simulink library "AEMS_Standard_Library"  (R2016b)
settings: Solver=ode45  StartTime=0.0  StopTime=10.0  RelTol=1e-3
undefined symbols (not defined in the file or in its folder): BkPY, carto, Cbx_extegr, Cbx_lpegrsys, Cbx_portegr, Cnx_bnk_nr_conf, Cnx_cyl_nr_conf, ConfigManagement, configuration_management, Cxx_dcm_io_tmr_end_xxxx, Cxx_dcm_rt_tmr_end, Cxx_DID_xxxx_IO_max, Cxx_DID_xxxx_IO_min, Cxx_egrhsofs, Cxx_vmaniegi, DEM_DEBOUNCE_FREEZE, DEM_DTR_CTL_INVISIBLE, DEM_DTR_CTL_NORMAL, Dem_DtrId2_XXX, Dem_DtrId3_XXX, Dem_DtrId4_XXX, Dem_DtrId5_XXX, Dem_DtrId6_XXX, Dem_DtrId7_XXX, Dem_DtrId8_XXX, Dem_DtrId9_XXX, Dem_DtrId_XXX, Dem_EnableConditionId2_XXX, Dem_EnableConditionId3_XXX, Dem_EnableConditionId4_XXX, Dem_EnableConditionId5_XXX, Dem_EnableConditionId6_XXX, Dem_EnableConditionId7_XXX, Dem_EnableConditionId8_XXX, Dem_EnableConditionId_XXX, Dem_EventId, Dem_EventId2_XXX, Dem_EventId3_XXX, Dem_EventId4_XXX, Dem_EventId5_XXX, Dem_EventId6_XXX, Dem_EventId7_XXX, Dem_EventId8_XXX, Dem_EventId9_XXX, Dem_EventId_Device_Faulttype, Dem_EventId_XXX, DEM_IUMPR_GENERAL_DENOMINATOR, DEM_OPCYC_IGNITION, Dem_RatioId2_XXX, Dem_RatioId3_XXX, Dem_RatioId4_XXX, Dem_RatioId5_XXX, Dem_RatioId6_XXX, Dem_RatioId7_XXX, Dem_RatioId8_XXX, Dem_RatioId_XXX, Dem_StorageConditionId2_XXX, Dem_StorageConditionId3_XXX, Dem_StorageConditionId4_XXX, Dem_StorageConditionId5_XXX ... (+65)
libraries: AEMS_Standard_Library x477, simulink x2
(part 27 of 39)

== system AEMS_Standard_Library/DISCONTINUITIES/AEMS_MULTI_PORT_TIME_SWITCH/pulse_and_old ==
  Vsx_sel : Inport  Tag=AM,In,0,1,Name,C;CMP,Port,PortWidth,SampleTime;
  AEMS_UNITDELAY_EXTERNALIC : AEMS_Standard_Library/DISCRETE/AEMS_UNITDELAY_EXTERNALIC  Tag=[LIB]
      settings: AttributesFormatString=%<MaskType>
  Relational_Operator : RelationalOperator  Tag=AM,Std,2,1;CMP,Operator;  Operator=~=  OutDataTypeStr=boolean  RndMeth=Nearest  InputSameDT=on
  Switch : Switch  Tag=GEN,Threshold;AM,Switch,2,1;CMP,Threshold;  Criteria=u2 ~= 0  RndMeth=Zero  SaturateOnIntegerOverflow=on  InputSameDT=on
      settings: AttributesFormatString=Criteria=%<Criteria>
  Unit_Delay : UnitDelay  Tag=GEN,X0,SampleTime;AM,Std,1,1;CMP,X0,SampleTime;  InitialCondition=1  SampleTime=-1
      settings: AttributesFormatString=IC = %<X0>
  Vbx_sel_puls : Outport  Tag=AM,Out,1,0,Name,NC;CMP,Port,OutputWhenDisabled,InitialOutput;
  Vsx_sel_old : Outport  Tag=AM,Out,1,0,Name,NC;CMP,Port,OutputWhenDisabled,InitialOutput;  Port=2
  wires:
  Unit_Delay/1 -> Switch/3
  Switch/1 -> Unit_Delay/1, Vsx_sel_old/1
  Relational_Operator/1 -> Switch/2, Vbx_sel_puls/1
  Vsx_sel/1 -> AEMS_UNITDELAY_EXTERNALIC/1, AEMS_UNITDELAY_EXTERNALIC/2, Relational_Operator/2
  AEMS_UNITDELAY_EXTERNALIC/1 -> Switch/1, Relational_Operator/1

== system AEMS_Standard_Library/DISCONTINUITIES/AEMS_MULTI_PORT_TIME_SWITCH/slop_on ==
  Vxx_swi_trs : Inport  Tag=AM,In,0,1,Name,C;CMP,Port,PortWidth,SampleTime;
  Vbx_sel_puls : Inport  Tag=AM,In,0,1,Name,C;CMP,Port,PortWidth,SampleTime;  Port=2
  Constant3 : Constant  Tag=AM,Constant,0,1,Value;CMP,Value;  OutDataTypeStr=Inherit: Inherit via back propagation
  Relational_Operator4 : RelationalOperator  Tag=AM,Std,2,1;CMP,Operator;  OutDataTypeStr=boolean  RndMeth=Nearest  InputSameDT=on
  SR_FlipFlop1 : Subsystem
  Terminator : Terminator
      settings: Tag=AM,Nothing;
  Vbx_slop_on : Outport  Tag=AM,Out,1,0,Name,NC;CMP,Port,OutputWhenDisabled,InitialOutput;
  wires:
  SR_FlipFlop1/2(QNot) -> Terminator/1
  SR_FlipFlop1/1(Q) -> Vbx_slop_on/1
  Vxx_swi_trs/1 -> Relational_Operator4/1
  Vbx_sel_puls/1 -> SR_FlipFlop1/1(S)
  Constant3/1 -> Relational_Operator4/2
  Relational_Operator4/1 -> SR_FlipFlop1/2(R)

== system AEMS_Standard_Library/DISCONTINUITIES/AEMS_MULTI_PORT_TIME_SWITCH/transient_timer ==
  Vxx_swi_t : Inport  Tag=AM,In,0,1,Name,C;CMP,Port,PortWidth,SampleTime;
  Vbx_sel_puls : Inport  Tag=AM,In,0,1,Name,C;CMP,Port,PortWidth,SampleTime;  Port=2
  dT : Inport  Tag=AM,In,0,1,Name,C;CMP,Port,PortWidth,SampleTime;  Port=3
  AEMS_DIVISION_BY_ZERO : Subsystem
  Constant1 : Constant  Tag=AM,Constant,0,1,Value;CMP,Value;  OutDataTypeStr=Inherit: Inherit via back propagation
  Constant2 : Constant  Tag=AM,Constant,0,1,Value;CMP,Value;  OutDataTypeStr=Inherit: Inherit via back propagation
  Constant4 : Constant  Tag=AM,Constant,0,1,Value;CMP,Value;  OutDataTypeStr=Inherit: Inherit via back propagation
  Relational_Operator3 : RelationalOperator  Tag=AM,Std,2,1;CMP,Operator;  OutDataTypeStr=boolean  RndMeth=Nearest  InputSameDT=on
  Sum : Sum  Tag=AM,Std,Inputs,1;CMP,Inputs;  OutDataTypeStr=Inherit: Inherit via back propagation  RndMeth=Zero  InputSameDT=on
  Switch : Switch  Tag=GEN,Threshold;AM,Switch,2,1;CMP,Threshold;  Criteria=u2 ~= 0  RndMeth=Zero  SaturateOnIntegerOverflow=on  InputSameDT=on
      settings: AttributesFormatString=Criteria=%<Criteria>
  Switch1 : Switch  Tag=GEN,Threshold;AM,Switch,2,1;CMP,Threshold;  Criteria=u2 ~= 0  RndMeth=Zero  SaturateOnIntegerOverflow=on  InputSameDT=on
      settings: AttributesFormatString=Criteria=%<Criteria>
  Unit_Delay1 : UnitDelay  Tag=GEN,X0,SampleTime;AM,Std,1,1;CMP,X0,SampleTime;  SampleTime=-1
      settings: AttributesFormatString=IC = %<X0>
  Vxx_swi_trs : Outport  Tag=AM,Out,1,0,Name,NC;CMP,Port,OutputWhenDisabled,InitialOutput;
  wires:
  Unit_Delay1/1 -> Sum/2, Relational_Operator3/1
  AEMS_DIVISION_BY_ZERO/1(ans) -> Sum/1, Switch/1
  Vbx_sel_puls/1 -> Switch/2
  Switch/1 -> Unit_Delay1/1, Vxx_swi_trs/1
  Sum/1 -> Switch1/3
  Switch1/1 -> Switch/3
  Constant1/1 -> Relational_Operator3/2
  Relational_Operator3/1 -> Switch1/2
  Constant2/1 -> Switch1/1
  Constant4/1 -> AEMS_DIVISION_BY_ZERO/3(ans_of_0div)
  dT/1 -> AEMS_DIVISION_BY_ZERO/2(num)
  Vxx_swi_t/1 -> AEMS_DIVISION_BY_ZERO/1(den)

== system AEMS_Standard_Library/DISCONTINUITIES/AEMS_SLEW_RATE/Slew_rate ==
  MAX_SLEW_RATE : Inport
  INPUT : Inport  Port=2
  MIN_SLEW_RATE : Inport  Port=3
  Constant1 : Constant  Value=true
  Slewing : Subsystem
  Switch : Switch  Criteria=u2 ~= 0  RndMeth=Zero  SaturateOnIntegerOverflow=on  InputSameDT=on
      settings: AttributesFormatString=Criteria=%<Criteria>
  UnitDelay : UnitDelay  SampleTime=-1
      settings: AttributesFormatString=IC = %<X0>
  UnitDelay1 : UnitDelay  InitialCondition=false  SampleTime=-1
      settings: AttributesFormatString=IC = %<X0>
  OUTPUT : Outport
  wires:
  MAX_SLEW_RATE/1 -> Slewing/2(MAX_SLEW_RATE)
  Switch/1 -> UnitDelay/1, OUTPUT/1
  INPUT/1 -> Slewing/4(INPUT), Switch/3
  Slewing/1(OUTPUT) -> Switch/1
  MIN_SLEW_RATE/1 -> Slewing/3(MIN_SLEW_RATE)
  Constant1/1 -> UnitDelay1/1
  UnitDelay/1 -> Slewing/1(OUTPUT_Prev)
  UnitDelay1/1 -> Switch/2

== system AEMS_Standard_Library/DISCONTINUITIES/AEMS_SLOPE_SWITCH/Signal_Change_Compute ==
  Switch_Cmd : Inport
  Relational_Operator : RelationalOperator  Operator=~=  OutDataTypeStr=boolean  RndMeth=Nearest  InputSameDT=on
  UnitDelay : UnitDelay  SampleTime=-1
      settings: AttributesFormatString=IC = %<X0>
  Signal_Change : Outport
  wires:
  Relational_Operator/1 -> Signal_Change/1
  Switch_Cmd/1 -> Relational_Operator/1, UnitDelay/1
  UnitDelay/1 -> Relational_Operator/2

== system AEMS_Standard_Library/DISCONTINUITIES/AEMS_SLOPE_SWITCH/Slope_On_Block ==
  Signal_Change : Inport  Tag=AM,In,0,1,Name,C;CMP,Port,PortWidth,SampleTime;
  Input : Inport  Tag=AM,In,0,1,Name,C;CMP,Port,PortWidth,SampleTime;  Port=2
  Pos_Slope : Inport  Tag=AM,In,0,1,Name,C;CMP,Port,PortWidth,SampleTime;  Port=3
  Neg_Slope : Inport  Tag=AM,In,0,1,Name,C;CMP,Port,PortWidth,SampleTime;  Port=4
  Prev_Output : Inport  Port=5
  Enable_Slope_On_Block : EnablePort
      settings: AttributesFormatString=StatesWhenEnabling: %<StatesWhenEnabling>
  Error_Due_To_High_Slope_Test : Subsystem
  Output_Comparision : Subsystem
  Output_Not_Equals_Input : Outport  Tag=AM,Out,1,0,Name,NC;CMP,Port,OutputWhenDisabled,InitialOutput;
  Output : Outport  Tag=AM,Out,1,0,Name,NC;CMP,Port,OutputWhenDisabled,InitialOutput;  Port=2
  wires:
  Error_Due_To_High_Slope_Test/1(Test_passed) -> Output_Comparision/1(Test_passed)
  Neg_Slope/1 -> Output_Comparision/5(Neg_Slope)
  Input/1 -> Output_Comparision/2(Input)
  Pos_Slope/1 -> Output_Comparision/3(Pos_Slope)
  Prev_Output/1 -> Output_Comparision/4(Prev_Output)
  Output_Comparision/2(Output) -> Output/1
  Output_Comparision/1(Output_Not_Equals_Input) -> Output_Not_Equals_Input/1
  Output_Comparision/3(RelOp2_out) -> Error_Due_To_High_Slope_Test/2(Output_Less_Than_Input)
  Output_Comparision/4(RelOp1_out) -> Error_Due_To_High_Slope_Test/3(Output_Greater_Than_Input)
  Signal_Change/1 -> Error_Due_To_High_Slope_Test/1(Signal_Change)

== system AEMS_Standard_Library/DISCONTINUITIES/AEMS_SLOPE_SWITCH/Slope_On_Compute ==
  Signal_Change : Inport  Tag=AM,In,0,1,Name,C;CMP,Port,PortWidth,SampleTime;
  Output_Not_Equals_Input : Inport  Tag=AM,In,0,1,Name,C;CMP,Port,PortWidth,SampleTime;  Port=2
  Constant1 : Constant  Value=false
  Constant3 : Constant  Value=true
  LogicalOperator : Logic  Operator=OR  OutDataTypeStr=boolean
  Switch2 : Switch  Tag=GEN,Threshold;AM,Switch,2,1;CMP,Threshold;  Criteria=u2 ~= 0  RndMeth=Zero  SaturateOnIntegerOverflow=on  InputSameDT=on
      settings: AttributesFormatString=Criteria=%<Criteria>
  UnitDelay1 : UnitDelay  InitialCondition=false  SampleTime=-1
      settings: AttributesFormatString=IC = %<X0>
  Slope_On : Outport  Tag=AM,Out,1,0,Name,NC;CMP,Port,OutputWhenDisabled,InitialOutput;
  wires:
  Switch2/1 -> LogicalOperator/2
  Constant1/1 -> Switch2/3
  Constant3/1 -> UnitDelay1/1
  UnitDelay1/1 -> Switch2/2
  Signal_Change/1 -> Switch2/1
  LogicalOperator/1 -> Slope_On/1
  Output_Not_Equals_Input/1 -> LogicalOperator/1

== system AEMS_Standard_Library/DISCONTINUITIES/AEMS_SLOPE_SWITCH_3INPUTS/Signal_Change_Compute ==
  Switch_Cmd : Inport
  Relational_Operator : RelationalOperator  Operator=~=  OutDataTypeStr=boolean  RndMeth=Nearest  InputSameDT=on
  UnitDelay : UnitDelay  SampleTime=-1
      settings: AttributesFormatString=IC = %<X0>
  Signal_Change : Outport
  wires:
  UnitDelay/1 -> Relational_Operator/2
  Switch_Cmd/1 -> UnitDelay/1, Relational_Operator/1
  Relational_Operator/1 -> Signal_Change/1

== system AEMS_Standard_Library/DISCONTINUITIES/AEMS_SLOPE_SWITCH_3INPUTS/Slope_On_Block ==
  Signal_Change : Inport  Tag=AM,In,0,1,Name,C;CMP,Port,PortWidth,SampleTime;
  Input : Inport  Tag=AM,In,0,1,Name,C;CMP,Port,PortWidth,SampleTime;  Port=2
  Pos_Slope : Inport  Tag=AM,In,0,1,Name,C;CMP,Port,PortWidth,SampleTime;  Port=3
  Neg_Slope : Inport  Tag=AM,In,0,1,Name,C;CMP,Port,PortWidth,SampleTime;  Port=4
  Prev_Output : Inport  Port=5
  Enable_Slope_On_Block : EnablePort
      settings: AttributesFormatString=StatesWhenEnabling: %<StatesWhenEnabling>
  Error_Due_To_High_Slope_Test : Subsystem
  Output_Comparision : Subsystem
  Output_Not_Equals_Input : Outport  Tag=AM,Out,1,0,Name,NC;CMP,Port,OutputWhenDisabled,InitialOutput;
  Output : Outport  Tag=AM,Out,1,0,Name,NC;CMP,Port,OutputWhenDisabled,InitialOutput;  Port=2
  wires:
  Signal_Change/1 -> Error_Due_To_High_Slope_Test/1(Signal_Change)
  Output_Comparision/4(RelOp1_out) -> Error_Due_To_High_Slope_Test/2(Output_Greater_Than_Input)
  Output_Comparision/3(RelOp2_out) -> Error_Due_To_High_Slope_Test/3(Output_Less_Than_Input)
  Output_Comparision/1(Output_Not_Equals_Input) -> Output_Not_Equals_Input/1
  Output_Comparision/2(Output) -> Output/1
  Error_Due_To_High_Slope_Test/1(Test_passed) -> Output_Comparision/1(Test_passed)
  Prev_Output/1 -> Output_Comparision/4(Prev_Output)
  Pos_Slope/1 -> Output_Comparision/3(Pos_Slope)
  Input/1 -> Output_Comparision/2(Input)
  Neg_Slope/1 -> Output_Comparision/5(Neg_Slope)

== system AEMS_Standard_Library/DISCONTINUITIES/AEMS_SLOPE_SWITCH_3INPUTS/Slope_On_Compute ==
  Signal_Change : Inport  Tag=AM,In,0,1,Name,C;CMP,Port,PortWidth,SampleTime;
  Output_Not_Equals_Input : Inport  Tag=AM,In,0,1,Name,C;CMP,Port,PortWidth,SampleTime;  Port=2
  Constant : Constant  Value=true
  Constant1 : Constant  Value=false
  Logical_Operator : Logic  Operator=OR  OutDataTypeStr=boolean
  Switch1 : Switch  Tag=GEN,Threshold;AM,Switch,2,1;CMP,Threshold;  Criteria=u2 ~= 0  RndMeth=Zero  SaturateOnIntegerOverflow=on  InputSameDT=on
      settings: AttributesFormatString=Criteria=%<Criteria>
  UnitDelay3 : UnitDelay  InitialCondition=false  SampleTime=-1
      settings: AttributesFormatString=IC = %<X0>
  Slope_On : Outport  Tag=AM,Out,1,0,Name,NC;CMP,Port,OutputWhenDisabled,InitialOutput;
  wires:
  Output_Not_Equals_Input/1 -> Logical_Operator/1
  Logical_Operator/1 -> Slope_On/1
  Constant/1 -> UnitDelay3/1
  UnitDelay3/1 -> Switch1/2
  Switch1/1 -> Logical_Operator/2
  Signal_Change/1 -> Switch1/1
  Constant1/1 -> Switch1/3

== system AEMS_Standard_Library/DISCONTINUITIES/AEMS_SLOPE_SWITCH_4INPUTS/Signal_Change_Compute ==
  Switch_Cmd : Inport
  Relational_Operator : RelationalOperator  Operator=~=  OutDataTypeStr=boolean  RndMeth=Nearest  InputSameDT=on
  UnitDelay : UnitDelay  SampleTime=-1
      settings: AttributesFormatString=IC = %<X0>
  Signal_Change : Outport
  wires:
  UnitDelay/1 -> Relational_Operator/2
  Switch_Cmd/1 -> UnitDelay/1, Relational_Operator/1
  Relational_Operator/1 -> Signal_Change/1

== system AEMS_Standard_Library/DISCONTINUITIES/AEMS_SLOPE_SWITCH_4INPUTS/Slope_On_Block ==
  Signal_Change : Inport  Tag=AM,In,0,1,Name,C;CMP,Port,PortWidth,SampleTime;
  Input : Inport  Tag=AM,In,0,1,Name,C;CMP,Port,PortWidth,SampleTime;  Port=2
  Pos_Slope : Inport  Tag=AM,In,0,1,Name,C;CMP,Port,PortWidth,SampleTime;  Port=3
  Neg_Slope : Inport  Tag=AM,In,0,1,Name,C;CMP,Port,PortWidth,SampleTime;  Port=4
  Prev_Output : Inport  Port=5
  Enable_Slope_On_Block : EnablePort
      settings: AttributesFormatString=StatesWhenEnabling: %<StatesWhenEnabling>
  Error_Due_To_High_Slope_Test : Subsystem
  Output_Comparision : Subsystem
  Output_Not_Equals_Input : Outport  Tag=AM,Out,1,0,Name,NC;CMP,Port,OutputWhenDisabled,InitialOutput;
  Output : Outport  Tag=AM,Out,1,0,Name,NC;CMP,Port,OutputWhenDisabled,InitialOutput;  Port=2
  wires:
  Signal_Change/1 -> Error_Due_To_High_Slope_Test/1(Signal_Change)
  Output_Comparision/4(RelOp1_out) -> Error_Due_To_High_Slope_Test/2(Output_Greater_Than_Input)
  Output_Comparision/3(RelOp2_out) -> Error_Due_To_High_Slope_Test/3(Output_Less_Than_Input)
  Output_Comparision/1(Output_Not_Equals_Input) -> Output_Not_Equals_Input/1
  Output_Comparision/2(Output) -> Output/1
  Error_Due_To_High_Slope_Test/1(Test_passed) -> Output_Comparision/1(Test_passed)
  Prev_Output/1 -> Output_Comparision/4(Prev_Output)
  Pos_Slope/1 -> Output_Comparision/3(Pos_Slope)
  Input/1 -> Output_Comparision/2(Input)
  Neg_Slope/1 -> Output_Comparision/5(Neg_Slope)

== system AEMS_Standard_Library/DISCONTINUITIES/AEMS_SLOPE_SWITCH_4INPUTS/Slope_On_Compute ==
  Signal_Change : Inport  Tag=AM,In,0,1,Name,C;CMP,Port,PortWidth,SampleTime;
  Output_Not_Equals_Input : Inport  Tag=AM,In,0,1,Name,C;CMP,Port,PortWidth,SampleTime;  Port=2
  Constant : Constant  Value=true
  Constant1 : Constant  Value=false
  Logical_Operator : Logic  Operator=OR  OutDataTypeStr=boolean
  Switch1 : Switch  Tag=GEN,Threshold;AM,Switch,2,1;CMP,Threshold;  Criteria=u2 ~= 0  RndMeth=Zero  SaturateOnIntegerOverflow=on  InputSameDT=on
      settings: AttributesFormatString=Criteria=%<Criteria>
  UnitDelay3 : UnitDelay  InitialCondition=false  SampleTime=-1
      settings: AttributesFormatString=IC = %<X0>
  Slope_On : Outport  Tag=AM,Out,1,0,Name,NC;CMP,Port,OutputWhenDisabled,InitialOutput;
  wires:
  Output_Not_Equals_Input/1 -> Logical_Operator/1
  Logical_Operator/1 -> Slope_On/1
  Constant/1 -> UnitDelay3/1
  UnitDelay3/1 -> Switch1/2
  Switch1/1 -> Logical_Operator/2
  Signal_Change/1 -> Switch1/1
  Constant1/1 -> Switch1/3

== system AEMS_Standard_Library/DISCONTINUITIES/AEMS_SLOPE_SWITCH_6INPUTS/Signal_Change_Compute ==
  Switch_Cmd : Inport
  Relational_Operator : RelationalOperator  Operator=~=  OutDataTypeStr=boolean  RndMeth=Nearest  InputSameDT=on
  Unit_Delay : UnitDelay  SampleTime=-1
      settings: AttributesFormatString=IC = %<X0>
  Signal_Change : Outport
  wires:
  Relational_Operator/1 -> Signal_Change/1
  Switch_Cmd/1 -> Relational_Operator/1, Unit_Delay/1
  Unit_Delay/1 -> Relational_Operator/2

== system AEMS_Standard_Library/DISCONTINUITIES/AEMS_SLOPE_SWITCH_6INPUTS/Slope_On_Block ==
  Signal_Change : Inport  Tag=AM,In,0,1,Name,C;CMP,Port,PortWidth,SampleTime;
  Input : Inport  Tag=AM,In,0,1,Name,C;CMP,Port,PortWidth,SampleTime;  Port=2
  Pos_Slope : Inport  Tag=AM,In,0,1,Name,C;CMP,Port,PortWidth,SampleTime;  Port=3
  Neg_Slope : Inport  Tag=AM,In,0,1,Name,C;CMP,Port,PortWidth,SampleTime;  Port=4
  Prev_Output : Inport  Port=5
  Enable_Slope_On_Block : EnablePort
      settings: AttributesFormatString=StatesWhenEnabling: %<StatesWhenEnabling>
  Error_Due_To_High_Slope_Test : Subsystem
  Output_Comparision : Subsystem
  Output_Not_Equals_Input : Outport  Tag=AM,Out,1,0,Name,NC;CMP,Port,OutputWhenDisabled,InitialOutput;
  Output : Outport  Tag=AM,Out,1,0,Name,NC;CMP,Port,OutputWhenDisabled,InitialOutput;  Port=2
  wires:
  Error_Due_To_High_Slope_Test/1(Test_passed) -> Output_Comparision/1(Test_passed)
  Neg_Slope/1 -> Output_Comparision/5(Neg_Slope)
  Input/1 -> Output_Comparision/2(Input)
  Pos_Slope/1 -> Output_Comparision/3(Pos_Slope)
  Prev_Output/1 -> Output_Comparision/4(Prev_Output)
  Output_Comparision/2(Output) -> Output/1
  Output_Comparision/1(Output_Not_Equals_Input) -> Output_Not_Equals_Input/1
  Output_Comparision/3(RelOp2_out) -> Error_Due_To_High_Slope_Test/2(Output_Less_Than_Input)
  Output_Comparision/4(RelOp1_out) -> Error_Due_To_High_Slope_Test/3(Output_Greater_Than_Input)
  Signal_Change/1 -> Error_Due_To_High_Slope_Test/1(Signal_Change)

== system AEMS_Standard_Library/DISCONTINUITIES/AEMS_SLOPE_SWITCH_6INPUTS/Slope_On_Compute ==
  Signal_Change : Inport  Tag=AM,In,0,1,Name,C;CMP,Port,PortWidth,SampleTime;
  Output_Not_Equals_Input : Inport  Tag=AM,In,0,1,Name,C;CMP,Port,PortWidth,SampleTime;  Port=2
  Constant : Constant  Value=true
  Constant1 : Constant  Value=false
  Logical_Operator : Logic  Operator=OR  OutDataTypeStr=boolean
  Switch1 : Switch  Tag=GEN,Threshold;AM,Switch,2,1;CMP,Threshold;  Criteria=u2 ~= 0  RndMeth=Zero  SaturateOnIntegerOverflow=on  InputSameDT=on
      settings: AttributesFormatString=Criteria=%<Criteria>
  Unit_Delay3 : UnitDelay  InitialCondition=false  SampleTime=-1
      settings: AttributesFormatString=IC = %<X0>
  Slope_On : Outport  Tag=AM,Out,1,0,Name,NC;CMP,Port,OutputWhenDisabled,InitialOutput;
  wires:
  Constant1/1 -> Switch1/3
  Signal_Change/1 -> Switch1/1
  Switch1/1 -> Logical_Operator/2
  Unit_Delay3/1 -> Switch1/2
  Constant/1 -> Unit_Delay3/1
  Logical_Operator/1 -> Slope_On/1
  Output_Not_Equals_Input/1 -> Logical_Operator/1

== system AEMS_Standard_Library/DISCONTINUITIES/AEMS_SLOPE_SWITCH_8INPUTS/Signal_Change_Compute ==
  Switch_Cmd : Inport
  Relational_Operator : RelationalOperator  Operator=~=  OutDataTypeStr=boolean  RndMeth=Nearest  InputSameDT=on
  Unit_Delay : UnitDelay  SampleTime=-1
      settings: AttributesFormatString=IC = %<X0>
  Signal_Change : Outport
  wires:
  Relational_Operator/1 -> Signal_Change/1
  Switch_Cmd/1 -> Relational_Operator/1, Unit_Delay/1
  Unit_Delay/1 -> Relational_Operator/2

== system AEMS_Standard_Library/DISCONTINUITIES/AEMS_SLOPE_SWITCH_8INPUTS/Slope_On_Block ==
  Signal_Change : Inport  Tag=AM,In,0,1,Name,C;CMP,Port,PortWidth,SampleTime;
  Input : Inport  Tag=AM,In,0,1,Name,C;CMP,Port,PortWidth,SampleTime;  Port=2
  Pos_Slope : Inport  Tag=AM,In,0,1,Name,C;CMP,Port,PortWidth,SampleTime;  Port=3
  Neg_Slope : Inport  Tag=AM,In,0,1,Name,C;CMP,Port,PortWidth,SampleTime;  Port=4
  Prev_Output : Inport  Port=5
  Enable_Slope_On_Block : EnablePort
      settings: AttributesFormatString=StatesWhenEnabling: %<StatesWhenEnabling>
  Error_Due_To_High_Slope_Test : Subsystem
  Output_Comparision : Subsystem
  Output_Not_Equals_Input : Outport  Tag=AM,Out,1,0,Name,NC;CMP,Port,OutputWhenDisabled,InitialOutput;
  Output : Outport  Tag=AM,Out,1,0,Name,NC;CMP,Port,OutputWhenDisabled,InitialOutput;  Port=2
  wires:
  Error_Due_To_High_Slope_Test/1(Test_passed) -> Output_Comparision/1(Test_passed)
  Neg_Slope/1 -> Output_Comparision/5(Neg_Slope)
  Input/1 -> Output_Comparision/2(Input)
  Pos_Slope/1 -> Output_Comparision/3(Pos_Slope)
  Prev_Output/1 -> Output_Comparision/4(Prev_Output)
  Output_Comparision/2(Output) -> Output/1
  Output_Comparision/1(Output_Not_Equals_Input) -> Output_Not_Equals_Input/1
  Output_Comparision/3(RelOp2_out) -> Error_Due_To_High_Slope_Test/2(Output_Less_Than_Input)
  Output_Comparision/4(RelOp1_out) -> Error_Due_To_High_Slope_Test/3(Output_Greater_Than_Input)
  Signal_Change/1 -> Error_Due_To_High_Slope_Test/1(Signal_Change)

== system AEMS_Standard_Library/DISCONTINUITIES/AEMS_SLOPE_SWITCH_8INPUTS/Slope_On_Compute ==
  Signal_Change : Inport  Tag=AM,In,0,1,Name,C;CMP,Port,PortWidth,SampleTime;
  Output_Not_Equals_Input : Inport  Tag=AM,In,0,1,Name,C;CMP,Port,PortWidth,SampleTime;  Port=2
  Constant : Constant  Value=true
  Constant1 : Constant  Value=false
  Logical_Operator : Logic  Operator=OR  OutDataTypeStr=boolean
  Switch1 : Switch  Tag=GEN,Threshold;AM,Switch,2,1;CMP,Threshold;  Criteria=u2 ~= 0  RndMeth=Zero  SaturateOnIntegerOverflow=on  InputSameDT=on
      settings: AttributesFormatString=Criteria=%<Criteria>
  Unit_Delay3 : UnitDelay  InitialCondition=false  SampleTime=-1
      settings: AttributesFormatString=IC = %<X0>
  Slope_On : Outport  Tag=AM,Out,1,0,Name,NC;CMP,Port,OutputWhenDisabled,InitialOutput;
  wires:
  Constant1/1 -> Switch1/3
  Signal_Change/1 -> Switch1/1
  Switch1/1 -> Logical_Operator/2
  Unit_Delay3/1 -> Switch1/2
  Constant/1 -> Unit_Delay3/1
  Logical_Operator/1 -> Slope_On/1
  Output_Not_Equals_Input/1 -> Logical_Operator/1

== system AEMS_Standard_Library/FILTER/AEMS_FILTER_WITH_DELAY_CONTROL/DivisionByZero ==
  ans_of_0div : Inport  Tag=AM,In,0,1,Name,C;CMP,Port,PortWidth,SampleTime;
  num : Inport  Tag=AM,In,0,1,Name,C;CMP,Port,PortWidth,SampleTime;  Port=2
  den : Inport  Tag=AM,In,0,1,Name,C;CMP,Port,PortWidth,SampleTime;  Port=3
  Divide : Product  Inputs=*/  OutDataTypeStr=Inherit: Inherit via back propagation  RndMeth=Zero
  MinMax1 : MinMax  Function=max  Inputs=2  OutDataTypeStr=Inherit: Inherit via back propagation  RndMeth=Zero  InputSameDT=on
  RelationalOperator : RelationalOperator  Tag=AM,Std,2,1;CMP,Operator;  Operator=~=  OutDataTypeStr=boolean  RndMeth=Nearest  InputSameDT=on
  Switch1 : Switch  Tag=GEN,Threshold;AM,Switch,2,1;CMP,Threshold;  Criteria=u2 ~= 0  RndMeth=Zero  SaturateOnIntegerOverflow=on  InputSameDT=on
      settings: AttributesFormatString=Criteria=%<Criteria>
  imm_zero : Constant  Tag=AM,Constant,0,1,Value;CMP,Value;  Value=0  OutDataTypeStr=Inherit: Inherit via back propagation
  imm_zero3 : Constant  Tag=AM,Constant,0,1,Value;CMP,Value;  Value=1.1920929e-07  OutDataTypeStr=Inherit: Inherit via back propagation
  ans : Outport  Tag=AM,Out,1,0,Name,NC;CMP,Port,OutputWhenDisabled,InitialOutput;
  wires:
  RelationalOperator/1 -> Switch1/2
  imm_zero/1 -> RelationalOperator/2
  Switch1/1 -> ans/1
  num/1 -> Divide/1
  Divide/1 -> Switch1/1
  ans_of_0div/1 -> Switch1/3
  den/1 -> RelationalOperator/1, MinMax1/2
  MinMax1/1 -> Divide/2
  imm_zero3/1 -> MinMax1/1

== system AEMS_Standard_Library/FILTER/AEMS_FILTER_WITH_DELAY_CONTROL/First_Order_Filter ==
  filter_parameter : Inport
      settings: AttributesFormatString=<tsample=%<SampleTime>>
  input : Inport  Port=2
      settings: AttributesFormatString=<tsample=%<SampleTime>>
  initial : Inport  Port=3  OutDataTypeStr=boolean
      settings: AttributesFormatString=<tsample=%<SampleTime>>
  Constant1 : Constant  OutDataTypeStr=Inherit: Inherit via back propagation
  Product : Product  SaturateOnIntegerOverflow=on  RndMeth=Zero
  Product1 : Product  SaturateOnIntegerOverflow=on  RndMeth=Zero
  Saturation : Saturate  UpperLimit=1  LowerLimit=0
      settings: AttributesFormatString=<limits=%<UpperLimit>/%<LowerLimit>>
  Sum : Sum  Inputs=-+  SaturateOnIntegerOverflow=on
  Sum1 : Sum  SaturateOnIntegerOverflow=on
  Switch1 : Switch  Threshold=0.5  SaturateOnIntegerOverflow=on  InputSameDT=on
      settings: AttributesFormatString=<threshold=%<threshold>>
  Unit Delay : UnitDelay  SampleTime=-1
      settings: AttributesFormatString=<initial=%<X0>>
  output : Outport
  wires:
  Saturation/1 -> Sum/1, Product/2  "limitted_fileter_parameter"
  Switch1/1 -> Unit Delay/1, output/1  "output"
  Product/1 -> Sum1/1
  Sum1/1 -> Switch1/3  "output"
  Product1/1 -> Sum1/2
  filter_parameter/1 -> Saturation/1
  initial/1 -> Switch1/2
  Unit Delay/1 -> Product1/2  "output_old"
  input/1 -> Product/1, Switch1/1
  Constant1/1 -> Sum/2
  Sum/1 -> Product1/1

== system AEMS_Standard_Library/FILTER/AEMS_FILTER_WITH_DELAY_CONTROL/First_Order_Filter1 ==
  filter_parameter : Inport
      settings: AttributesFormatString=<tsample=%<SampleTime>>
  input : Inport  Port=2
      settings: AttributesFormatString=<tsample=%<SampleTime>>
  initial : Inport  Port=3  OutDataTypeStr=boolean
      settings: AttributesFormatString=<tsample=%<SampleTime>>
  Constant1 : Constant  OutDataTypeStr=Inherit: Inherit via back propagation
  Product : Product  SaturateOnIntegerOverflow=on  RndMeth=Zero
  Product1 : Product  SaturateOnIntegerOverflow=on  RndMeth=Zero
  Saturation : Saturate  UpperLimit=1  LowerLimit=0
      settings: AttributesFormatString=<limits=%<UpperLimit>/%<LowerLimit>>
  Sum : Sum  Inputs=-+  SaturateOnIntegerOverflow=on
  Sum1 : Sum  SaturateOnIntegerOverflow=on
  Switch1 : Switch  Threshold=0.5  SaturateOnIntegerOverflow=on  InputSameDT=on
      settings: AttributesFormatString=<threshold=%<threshold>>
  Unit Delay : UnitDelay  SampleTime=-1
      settings: AttributesFormatString=<initial=%<X0>>
  output : Outport
  wires:
  Sum/1 -> Product1/1
  Constant1/1 -> Sum/2
  input/1 -> Switch1/1, Product/1
  Unit Delay/1 -> Product1/2  "output_old"
  initial/1 -> Switch1/2
  filter_parameter/1 -> Saturation/1
  Product1/1 -> Sum1/2
  Sum1/1 -> Switch1/3  "output"
  Product/1 -> Sum1/1
  Switch1/1 -> output/1, Unit Delay/1  "output"
  Saturation/1 -> Product/2, Sum/1  "limitted_fileter_parameter"

== system AEMS_Standard_Library/FILTER/AEMS_FILTER_WITH_DELAY_CONTROL/First_Order_Filter2 ==
  filter_parameter : Inport
      settings: AttributesFormatString=<tsample=%<SampleTime>>
  input : Inport  Port=2
      settings: AttributesFormatString=<tsample=%<SampleTime>>
  initial : Inport  Port=3  OutDataTypeStr=boolean
      settings: AttributesFormatString=<tsample=%<SampleTime>>
  Constant1 : Constant  OutDataTypeStr=Inherit: Inherit via back propagation
  Product : Product  SaturateOnIntegerOverflow=on  RndMeth=Zero
  Product1 : Product  SaturateOnIntegerOverflow=on  RndMeth=Zero
  Saturation : Saturate  UpperLimit=1  LowerLimit=0
      settings: AttributesFormatString=<limits=%<UpperLimit>/%<LowerLimit>>
  Sum : Sum  Inputs=-+  SaturateOnIntegerOverflow=on
  Sum1 : Sum  SaturateOnIntegerOverflow=on
  Switch1 : Switch  Threshold=0.5  SaturateOnIntegerOverflow=on  InputSameDT=on
      settings: AttributesFormatString=<threshold=%<threshold>>
  Unit Delay : UnitDelay  SampleTime=-1
      settings: AttributesFormatString=<initial=%<X0>>
  output : Outport
  wires:
  Saturation/1 -> Sum/1, Product/2  "limitted_fileter_parameter"
  Switch1/1 -> Unit Delay/1, output/1  "output"
  Product/1 -> Sum1/1
  Sum1/1 -> Switch1/3  "output"
  Product1/1 -> Sum1/2
  filter_parameter/1 -> Saturation/1
  initial/1 -> Switch1/2
  Unit Delay/1 -> Product1/2  "output_old"
  input/1 -> Product/1, Switch1/1
  Constant1/1 -> Sum/2
  Sum/1 -> Product1/1

== system AEMS_Standard_Library/LOOKUP_TABLES/AEMS_INDEXED_LUT_1D_TOL/PreLookUpX ==
  u : Inport
  Constant1 : Constant
  Constant3 : Constant
  Data Type Conversion : DataTypeConversion  OutDataTypeStr=uint32
  MinMax : MinMax  Function=max  Inputs=2
  Relational Operator : RelationalOperator  OutDataTypeStr=boolean  RndMeth=Nearest  InputSameDT=on
  Sum of Elements : Sum  Inputs=+-
  Sum of Elements1 : Sum  Inputs=+
  X_Tolerance2 : Constant  Value=map_x
  k : Outport
  wires:
  Data Type Conversion/1 -> Sum of Elements1/1
  X_Tolerance2/1 -> Relational Operator/2
  u/1 -> Relational Operator/1
  Constant3/1 -> MinMax/2
  Constant1/1 -> Sum of Elements/2
  MinMax/1 -> Sum of Elements/1
  Sum of Elements/1 -> k/1
  Relational Operator/1 -> Data Type Conversion/1
  Sum of Elements1/1 -> MinMax/1

== system AEMS_Standard_Library/LOOKUP_TABLES/AEMS_INDEXED_LUT_1D_TOL/PreLookUpX+Tol ==
  u : Inport
  Constant1 : Constant
  Constant3 : Constant
  Data Type Conversion : DataTypeConversion  OutDataTypeStr=uint32
  MinMax : MinMax  Function=max  Inputs=2
  Relational Operator : RelationalOperator  OutDataTypeStr=boolean  RndMeth=Nearest  InputSameDT=on
  Sum of Elements : Sum  Inputs=+-
  Sum of Elements1 : Sum  Inputs=+
  X_Tolerance2 : Constant  Value=map_x
  k : Outport
  wires:
  Data Type Conversion/1 -> Sum of Elements1/1
  X_Tolerance2/1 -> Relational Operator/2
  u/1 -> Relational Operator/1
  Constant3/1 -> MinMax/2
  Constant1/1 -> Sum of Elements/2
  MinMax/1 -> Sum of Elements/1
  Sum of Elements/1 -> k/1
  Relational Operator/1 -> Data Type Conversion/1
  Sum of Elements1/1 -> MinMax/1

== system AEMS_Standard_Library/LOOKUP_TABLES/AEMS_INDEXED_LUT_2D_TOL/PreLookUpX ==
  u : Inport
  " " : DataTypeConversion  OutDataTypeStr=uint32
  Constant1 : Constant
  Constant3 : Constant
  MinMax : MinMax  Function=max  Inputs=2
  Relational Operator : RelationalOperator  OutDataTypeStr=boolean  RndMeth=Nearest
  Sum of Elements : Sum  Inputs=+-
  Sum of Elements1 : Sum  Inputs=+
  X_Tolerance2 : Constant  Tag=AM,Constant,0,1,Value;CMP,Value;  Value=map_x
  k : Outport
  wires:
  " "/1 -> Sum of Elements1/1
  X_Tolerance2/1 -> Relational Operator/2
  u/1 -> Relational Operator/1
  Constant3/1 -> MinMax/2
  Constant1/1 -> Sum of Elements/2
  MinMax/1 -> Sum of Elements/1
  Sum of Elements/1 -> k/1
  Relational Operator/1 -> " "/1
  Sum of Elements1/1 -> MinMax/1

== system AEMS_Standard_Library/LOOKUP_TABLES/AEMS_INDEXED_LUT_2D_TOL/PreLookUpX+Tol ==
  u : Inport
  " " : DataTypeConversion  OutDataTypeStr=uint32
  Constant1 : Constant
  Constant3 : Constant
  MinMax : MinMax  Function=max  Inputs=2
  Relational Operator : RelationalOperator  OutDataTypeStr=boolean  RndMeth=Nearest
  Sum of Elements : Sum  Inputs=+-
  Sum of Elements1 : Sum  Inputs=+
  X_Tolerance2 : Constant  Tag=AM,Constant,0,1,Value;CMP,Value;  Value=map_x
  k : Outport
  wires:
  " "/1 -> Sum of Elements1/1
  X_Tolerance2/1 -> Relational Operator/2
  u/1 -> Relational Operator/1
  Constant3/1 -> MinMax/2
  Constant1/1 -> Sum of Elements/2
  MinMax/1 -> Sum of Elements/1
  Sum of Elements/1 -> k/1
  Relational Operator/1 -> " "/1
  Sum of Elements1/1 -> MinMax/1

== system AEMS_Standard_Library/LOOKUP_TABLES/AEMS_INDEXED_LUT_2D_TOL/PreLookUpY ==
  u : Inport
  " " : DataTypeConversion  OutDataTypeStr=uint32
  Constant1 : Constant
  Constant3 : Constant
  MinMax : MinMax  Function=max  Inputs=2
  Relational Operator : RelationalOperator  OutDataTypeStr=boolean  RndMeth=Nearest
  Sum of Elements : Sum  Inputs=+-
  Sum of Elements1 : Sum  Inputs=+
  X_Tolerance2 : Constant  Tag=AM,Constant,0,1,Value;CMP,Value;  Value=map_y
  k : Outport
  wires:
  " "/1 -> Sum of Elements1/1
  X_Tolerance2/1 -> Relational Operator/2
  u/1 -> Relational Operator/1
  Constant3/1 -> MinMax/2
  Constant1/1 -> Sum of Elements/2
  MinMax/1 -> Sum of Elements/1
  Sum of Elements/1 -> k/1
  Relational Operator/1 -> " "/1
  Sum of Elements1/1 -> MinMax/1

== system AEMS_Standard_Library/LOOKUP_TABLES/AEMS_INDEXED_LUT_2D_TOL/PreLookUpY+Tol1 ==
  u : Inport
  " " : DataTypeConversion  OutDataTypeStr=uint32
  Constant1 : Constant
  Constant3 : Constant
  MinMax : MinMax  Function=max  Inputs=2
  Relational Operator : RelationalOperator  OutDataTypeStr=boolean  RndMeth=Nearest
  Sum of Elements : Sum  Inputs=+-
  Sum of Elements1 : Sum  Inputs=+
  X_Tolerance2 : Constant  Tag=AM,Constant,0,1,Value;CMP,Value;  Value=map_y
  k : Outport
  wires:
  Sum of Elements1/1 -> MinMax/1
  Relational Operator/1 -> " "/1
  Sum of Elements/1 -> k/1
  MinMax/1 -> Sum of Elements/1
  Constant1/1 -> Sum of Elements/2
  Constant3/1 -> MinMax/2
  u/1 -> Relational Operator/1
  X_Tolerance2/1 -> Relational Operator/2
  " "/1 -> Sum of Elements1/1

== system AEMS_Standard_Library/MATH/AEMS_IGN_TO_PHY/Inverse_order ==
  Order_vector : Inport
  Enable : EnablePort
      settings: AttributesFormatString=<states=%<StatesWhenEnabling>>
  Constant4 : Constant  OutDataTypeStr=Inherit: Inherit via back propagation
  Constant5 : Constant  Value=2  OutDataTypeStr=Inherit: Inherit via back propagation
  Constant6 : Constant  Value=3  OutDataTypeStr=Inherit: Inherit via back propagation
  Constant7 : Constant  Value=4  OutDataTypeStr=Inherit: Inherit via back propagation
  Constant8 : Constant  Value=5  OutDataTypeStr=Inherit: Inherit via back propagation
  Constant9 : Constant  Value=6  OutDataTypeStr=Inherit: Inherit via back propagation
  Mux2 : Mux  Inputs=6
  Subsystem1 : Subsystem
  Subsystem2 : Subsystem
  Subsystem3 : Subsystem
  Subsystem4 : Subsystem
  Subsystem5 : Subsystem
  Subsystem6 : Subsystem
  Inverted_vector : Outport
  wires:
  Constant6/1 -> Subsystem3/1(In)
  Subsystem3/1(Out) -> Mux2/3
  Constant4/1 -> Subsystem2/1(In)
  Subsystem6/1(Out) -> Mux2/6
  Subsystem4/1(Out) -> Mux2/4
  Subsystem1/1(Out) -> Mux2/2
  Subsystem2/1(Out) -> Mux2/1
  Subsystem5/1(Out) -> Mux2/5
  Constant5/1 -> Subsystem1/1(In)
  Constant7/1 -> Subsystem4/1(In)
  Constant8/1 -> Subsystem5/1(In)
  Constant9/1 -> Subsystem6/1(In)
  Order_vector/1 -> Subsystem6/2(Order_vector), Subsystem5/2(Order_vector), Subsystem4/2(Order_vector), Subsystem3/2(Order_vector), Subsystem1/2(Order_vector), Subsystem2/2(Order_vector)
  Mux2/1 -> Inverted_vector/1

== system AEMS_Standard_Library/MATH/AEMS_MATRIX_INVERSION/Co-factors of the Matrix ==
  m00 : Inport
  m01 : Inport  Port=2
  m02 : Inport  Port=3
  m10 : Inport  Port=4
  m11 : Inport  Port=5
  m12 : Inport  Port=6
  m21 : Inport  Port=7
  m22 : Inport  Port=8
  m23 : Inport  Port=9
  Co_m00 : Inport  Port=10
  Co_m10 : Inport  Port=11
  Co_m20 : Inport  Port=12
  Add{,1..5} (6 alike) : Sum  Inputs=+-  OutDataTypeStr=Inherit: Inherit via back propagation  SaturateOnIntegerOverflow=on  InputSameDT=on
  Gain{,1..3} (4 alike) : Gain  Gain=-1
  Mux2 : Mux  Inputs=3
  Mux3 : Mux  Inputs=3
  Mux4 : Mux  Inputs=3
  Product{1..12} (12 alike) : Product  OutDataTypeStr=Inherit: Inherit via back propagation
  Vector Concatenate : Concatenate  NumInputs=3  Mode=Multidimensional array  ConcatenateDimension=2
  Adj_m : Outport
  wires:
  Product1/1 -> Add/1
  Product2/1 -> Add/2
  Product3/1 -> Add1/1
  Product4/1 -> Add1/2
  Product5/1 -> Add2/1
  Product6/1 -> Add2/2
  Product7/1 -> Add3/1
  Product8/1 -> Add3/2
  Product9/1 -> Add4/1
  Product10/1 -> Add4/2
  Product11/1 -> Add5/1
  Product12/1 -> Add5/2
  Add/1 -> Gain1/1
  Add2/1 -> Gain2/1
  Add4/1 -> Gain3/1
  Add5/1 -> Mux4/3
  Vector Concatenate/1 -> Adj_m/1
  Mux2/1 -> Vector Concatenate/1
  Mux3/1 -> Vector Concatenate/2
  Mux4/1 -> Vector Concatenate/3
  Gain3/1 -> Mux4/2
  Add3/1 -> Mux4/1
  Gain2/1 -> Mux3/3
  Gain1/1 -> Mux3/1
  Gain/1 -> Mux2/2
  m00/1 -> Product11/1, Product9/1, Product5/1, Product3/1
  m01/1 -> Product1/1, Product12/1, Product7/1, Product6/1
  m02/1 -> Product10/1, Product8/1, Product4/1, Product2/1
  m23/1 -> Product1/2, Product3/2
  m22/1 -> Product2/2, Product5/2
  m21/1 -> Product6/2, Product4/2
  m12/1 -> Product9/2, Product7/2
  m11/1 -> Product8/2, Product11/2
  m10/1 -> Product10/2, Product12/2
  Add1/1 -> Mux3/2
  Co_m20/1 -> Mux2/3
  Co_m10/1 -> Gain/1
  Co_m00/1 -> Mux2/1

== system AEMS_Standard_Library/MATH/AEMS_MATRIX_INVERSION/Determinant of the Matrix ==
  m00 : Inport
  m01 : Inport  Port=2
  m02 : Inport  Port=3
  m10 : Inport  Port=4
  m11 : Inport  Port=5
  m12 : Inport  Port=6
  m20 : Inport  Port=7
  m21 : Inport  Port=8
  m22 : Inport  Port=9
  Add : Sum  Inputs=+-  OutDataTypeStr=Inherit: Inherit via back propagation  SaturateOnIntegerOverflow=on  InputSameDT=on
  Add1 : Sum  Inputs=+-  OutDataTypeStr=Inherit: Inherit via back propagation  SaturateOnIntegerOverflow=on  InputSameDT=on
  Add2 : Sum  Inputs=+-  OutDataTypeStr=Inherit: Inherit via back propagation  SaturateOnIntegerOverflow=on  InputSameDT=on
  Add5 : Sum  Inputs=+-+  OutDataTypeStr=Inherit: Inherit via back propagation  SaturateOnIntegerOverflow=on  InputSameDT=on
  Product{,1..8} (9 alike) : Product  OutDataTypeStr=Inherit: Inherit via back propagation
  Det_m : Outport
  Co_m11 : Outport  Port=2
  Co_m12 : Outport  Port=3
  Co_m13 : Outport  Port=4
  wires:
  m11/1 -> Product8/2, Product3/2
  m20/1 -> Product8/1, Product6/2
  m02/1 -> Product2/1
  m00/1 -> Product/1
  m21/1 -> Product4/2, Product7/2
  m12/1 -> Product6/1, Product4/1
  m10/1 -> Product7/1, Product5/2
  Product5/1 -> Add1/1
  Product3/1 -> Add/1
  Product1/1 -> Add5/2
  Add1/1 -> Product1/2, Co_m12/1
  Product/1 -> Add5/1
  Add/1 -> Product/2, Co_m11/1
  Product2/1 -> Add5/3
  Product6/1 -> Add1/2
  Product7/1 -> Add2/1
  Add5/1 -> Det_m/1
  Add2/1 -> Product2/2, Co_m13/1
  Product4/1 -> Add/2
  Product8/1 -> Add2/2
  m01/1 -> Product1/1
  m22/1 -> Product5/1, Product3/1

== system AEMS_Standard_Library/MATH/AEMS_MATRIX_INVERSION/Elements of the Matrix ==
  m_3x3 : Inport
  Demux : Demux  Outputs=9
  Mux : Mux  Inputs=3
  Selector1 : Selector  NumberOfDimensions=2  InputPortWidth=10  IndexOptions=Starting index (dialog),Index vector (dialog)  Indices=2,[1 2 3]  OutputSizes=1,1
  Selector2 : Selector  NumberOfDimensions=2  InputPortWidth=10  IndexOptions=Starting index (dialog),Index vector (dialog)  Indices=1,[1 2 3]  OutputSizes=1,1
  Selector9 : Selector  NumberOfDimensions=2  InputPortWidth=10  IndexOptions=Starting index (dialog),Index vector (dialog)  Indices=3,[1 2 3]  OutputSizes=1,1
  m00 : Outport
  m01 : Outport  Port=2
  m02 : Outport  Port=3
  m10 : Outport  Port=4
  m11 : Outport  Port=5
  m12 : Outport  Port=6
  m20 : Outport  Port=7
  m21 : Outport  Port=8
  m22 : Outport  Port=9
  wires:
  m_3x3/1 -> Selector2/1, Selector9/1, Selector1/1
  Selector1/1 -> Mux/2
  Selector9/1 -> Mux/3
  Selector2/1 -> Mux/1
  Mux/1 -> Demux/1
  Demux/9 -> m22/1
  Demux/6 -> m12/1
  Demux/5 -> m11/1
  Demux/8 -> m21/1
  Demux/7 -> m20/1
  Demux/2 -> m01/1
  Demux/1 -> m00/1
  Demux/3 -> m02/1
  Demux/4 -> m10/1

== system AEMS_Standard_Library/MATH/AEMS_MATRIX_INVERSION/Matrix_inversion ==
  Adj_m : Inport
  Det_m : Inport  Port=2
  Alternate_Input : Inport  Port=3
  Action Port : ActionPort
  AEMS_PROTECTED_DIVISION : AEMS_Standard_Library/MATH/AEMS_PROTECTED_DIVISION  Tag=[LIB]  out_mode=Default_Output -> Output  tolerance=0.01
      settings: AttributesFormatString=%<MaskType>\nOutput when |Denominator| < Tolerance = %<out_mode>\nDenominator Tolerance = %<tolerance>
  Constant : Constant  OutDataTypeStr=Inherit: Inherit via back propagation
  Product : Product  OutDataTypeStr=Inherit: Inherit via back propagation
  " Inverted_Matrix" : Outport
  wires:
  AEMS_PROTECTED_DIVISION/1 -> Product/2
  Constant/1 -> AEMS_PROTECTED_DIVISION/1
  Alternate_Input/1 -> AEMS_PROTECTED_DIVISION/3
  Adj_m/1 -> Product/1
  Det_m/1 -> AEMS_PROTECTED_DIVISION/2
  Product/1 -> " Inverted_Matrix"/1

== system AEMS_Standard_Library/MATH/AEMS_MATRIX_INVERSION/Matrix_inversion_not_possible ==
  Alternate_Input : Inport
  Action Port : ActionPort
  " Alternate_Output" : Outport
  wires:
  Alternate_Input/1 -> " Alternate_Output"/1

== system AEMS_Standard_Library/MATH/AEMS_SORT/For_loop_1 ==
  Vector_to_sort : Inport
  Selected_index : Inport  Port=2
  Add : Sum  Inputs=-+  InputSameDT=on
  DataTypeConversion3 : DataTypeConversion  RndMeth=Zero
  For Iterator : ForIterator  IterationSource=external  IndexMode=Zero-based  IterationVariableDataType=int8
  For_loop_2 : Subsystem  TreatAsAtomicUnit=on
  Sorted_vector : Outport
  wires:
  Selected_index/1 -> For Iterator/1, Add/2
  For Iterator/1 -> DataTypeConversion3/1
  DataTypeConversion3/1 -> Add/1
  Add/1 -> For_loop_2/1(Index_loop)
  Vector_to_sort/1 -> For_loop_2/2(Vector_to_sort)
  For_loop_2/1("Sorted_vector ") -> Sorted_vector/1

== system AEMS_Standard_Library/SPECIFIC/AEMS_AIR_BALANCE/MWI_Cyl_Charge_Mass_Air_N ==
  rpm : Inport  Interpolate=off
  vcyl : Inport  Port=2  Interpolate=off
  egclrt : Inport  Port=3  Interpolate=off
  qcylegr_p : Inport  Port=4  Interpolate=off
  vmani : Inport  Port=5  Interpolate=off
  mamani : Inport  Port=6  Interpolate=off
  60*10^-1 : Constant  Value=0.00694  OutDataTypeStr=single
  60*10^-3 : Constant  Value=60  OutDataTypeStr=single
  Constant1 : Constant  OutDataTypeStr=single
  Constant2 : Constant  OutDataTypeStr=single
  Constant4 : Constant  Value=Cnx_cyl_nr_conf
  Gain : Gain  Gain=1000  ParamDataTypeStr=single  SaturateOnIntegerOverflow=on
  Gain1 : Gain  Gain=0.5  ParamDataTypeStr=single  SaturateOnIntegerOverflow=on
  MinMax : MinMax  Function=max  Inputs=2  SaturateOnIntegerOverflow=on  InputSameDT=on
  MinMax1 : MinMax  Function=max  Inputs=2  SaturateOnIntegerOverflow=on  InputSameDT=on
  Product{,3..7,9} (7 alike) : Product  SaturateOnIntegerOverflow=on  RndMeth=Zero  InputSameDT=on
  Product1 : Product  Inputs=*/  SaturateOnIntegerOverflow=on  RndMeth=Zero  InputSameDT=on
  Product2 : Product  Inputs=*/  SaturateOnIntegerOverflow=on  RndMeth=Zero  InputSameDT=on
  Product8 : Product  Inputs=*/  SaturateOnIntegerOverflow=on  RndMeth=Zero  InputSameDT=on
  Sum1 : Sum  Inputs=-+  SaturateOnIntegerOverflow=on  InputSameDT=on
  Sum2 : Sum  Inputs=-+  SaturateOnIntegerOverflow=on  InputSameDT=on
  Sum3 : Sum  SaturateOnIntegerOverflow=on  InputSameDT=on
  Switch2 : Switch  Criteria=u2 ~= 0  SaturateOnIntegerOverflow=on  InputSameDT=on
      settings: AttributesFormatString=Criteria=%<Criteria>
  mVMANI1 : Constant  Value=0.000001  OutDataTypeStr=single
  mVMANI2 : Constant  Value=Cxx_vmaniegi
  mVMANI4 : Constant  Value=Cbx_portegr
  qcyl : Outport
  qcylegr : Outport  Port=2
  qcylall : Outport  Port=3
  macyllj : Outport  Port=4
  egclrt_p : Outport  Port=5
  wires:
  Constant2/1 -> Sum2/2
  Sum2/1 -> Product9/1
  egclrt/1 -> Sum1/1, Product6/1
  Product9/1 -> Switch2/1
  Product7/1 -> Switch2/3  "macyllj"
  mVMANI4/1 -> Switch2/2
  Switch2/1 -> macyllj/1  "macyllj"
  qcylegr_p/1 -> Product8/1
  MinMax1/1 -> Product8/2
  60*10^-1/1 -> MinMax1/2
  Gain1/1 -> Product3/1  "tmp_nref"
  Constant4/1 -> Gain1/1
  Product6/1 -> qcylegr/1  "qcylegr"
  Product5/1 -> qcyl/1  "qcyl"
  Product8/1 -> Sum2/1, egclrt_p/1  "egclrt_p"
  Sum1/1 -> Product7/2, Product5/2  "airclrt"
  Constant1/1 -> Sum1/2
  Sum3/1 -> MinMax/1
  vmani/1 -> Sum3/2
  mVMANI2/1 -> Sum3/1
  MinMax/1 -> Product1/2
  mVMANI1/1 -> MinMax/2
  Product1/1 -> Product4/2, Gain/1  "mcylall_pm"
  Product3/1 -> Product6/2, qcylall/1, Product5/1, MinMax1/1  "qcylall"
  rpm/1 -> Product4/1
  60*10^-3/1 -> Product2/2
  Product4/1 -> Product2/1
  Product2/1 -> Product3/2
  vcyl/1 -> Product/2
  Product/1 -> Product1/1
  mamani/1 -> Product/1
  Gain/1 -> Product9/2, Product7/1

== system AEMS_Standard_Library/SPECIFIC/AEMS_AIR_BALANCE/MWI_Mani_Charge_Mass_Air_EGR ==
  tanmnp : Inport  Interpolate=off
  fqselgo : Inport  Port=2  Interpolate=off
  pargeqd : Inport  Port=3  Interpolate=off
  qegrve : Inport  Port=4  Interpolate=off
  ppamb : Inport  Port=5  Interpolate=off
  qtrm : Inport  Port=6  Interpolate=off
  qegrth : Inport  Port=7  Interpolate=off
  fafmlmsta : Inport  Port=8  Interpolate=off
  vmani : Inport  Port=9  Interpolate=off
  fair_egrv : Inport  Port=10  Interpolate=off
  qcyl_pudt : Inport  Port=11  Interpolate=off
  qcylegr_pudt : Inport  Port=12  Interpolate=off
  qcylall_pudt : Inport  Port=13  Interpolate=off
  EGRMANI_permission : Subsystem
  MWI_egrmani_pm_cal : Subsystem  Description=|
      | EGR mass of correcter is calculated.                               
      | EGR mass of correcter                                              
      | = integral (EGR coming into correcter - EGR going out of correcter)
  MWI_mamani_pm_cal : Subsystem  Description=|
      | Air mass and (air + EGR) mass of correcter is calculated.          
      | Air mass of correcter                                              
      | = integral (air coming into correcter - air going out of correcter)
  mamani : Outport
  airmani : Outport  Port=2
  egrmani : Outport  Port=3
  wires:
  vmani/1 -> MWI_mamani_pm_cal/11(vmani)
  fafmlmsta/1 -> MWI_mamani_pm_cal/10(fafmlmsta)
  EGRMANI_permission/1(egrmani_cal_ok) -> MWI_egrmani_pm_cal/Enable
  qcyl_pudt/1 -> MWI_mamani_pm_cal/8(qcyl_pudt)
  qtrm/1 -> MWI_mamani_pm_cal/7(qtrm)
  ppamb/1 -> MWI_mamani_pm_cal/6(ppamb)
  tanmnp/1 -> MWI_mamani_pm_cal/5(tanmnp)
  pargeqd/1 -> MWI_mamani_pm_cal/4(pargeqd)
  fqselgo/1 -> MWI_mamani_pm_cal/3(fqselgo)
  qegrth/1 -> MWI_mamani_pm_cal/2(qegrth)
  qcylall_pudt/1 -> MWI_mamani_pm_cal/9(qcylall_pudt)
  qegrve/1 -> MWI_egrmani_pm_cal/3(qegrve), MWI_mamani_pm_cal/12(qegrve)
  qcylegr_pudt/1 -> MWI_egrmani_pm_cal/1(qcylegr_pudt)
  MWI_egrmani_pm_cal/1(egrmani) -> MWI_mamani_pm_cal/1(egrmani), egrmani/1
  MWI_mamani_pm_cal/2(airmani) -> airmani/1
  MWI_mamani_pm_cal/1(mamani) -> mamani/1
  fair_egrv/1 -> MWI_egrmani_pm_cal/2(fair_egrv), MWI_mamani_pm_cal/13(fair_egrv)

== system AEMS_Standard_Library/SPECIFIC/AEMS_AIR_BALANCE/MWI_Manifold_Pressure_N ==
  vmani : Inport  Interpolate=off
  tanmnp : Inport  Port=2  Interpolate=off
  airmani : Inport  Port=3  Interpolate=off
  egrmani : Inport  Port=4  Interpolate=off
  Gain1 : Gain  Gain=0.00028704  ParamDataTypeStr=single  SaturateOnIntegerOverflow=on
  Gain2 : Gain  Gain=0.0002834  ParamDataTypeStr=single  SaturateOnIntegerOverflow=on
  MinMax : MinMax  Function=max  Inputs=2  SaturateOnIntegerOverflow=on  InputSameDT=on
  MinMax3 : MinMax  Function=max  Inputs=2  SaturateOnIntegerOverflow=on  InputSameDT=on
  Product5 : Product  Inputs=/*  SaturateOnIntegerOverflow=on  RndMeth=Zero  InputSameDT=on
  Product6 : Product  SaturateOnIntegerOverflow=on  RndMeth=Zero  InputSameDT=on
  Sum : Sum  SaturateOnIntegerOverflow=on  InputSameDT=on
  Sum1 : Sum  SaturateOnIntegerOverflow=on  InputSameDT=on
  Sum2 : Sum  SaturateOnIntegerOverflow=on  InputSameDT=on
  constant1 : Constant  Value=273  OutDataTypeStr=single
  constant4 : Constant  Value=10  OutDataTypeStr=single
  mVMANI1 : Constant  Value=0.000001  OutDataTypeStr=single
  mVMANI2 : Constant  Value=Cxx_vmaniegi
  pmani : Outport
  wires:
  MinMax3/1 -> pmani/1  "pmani"
  constant4/1 -> MinMax3/1
  Sum2/1 -> Product6/2
  Gain2/1 -> Sum2/2
  Gain1/1 -> Sum2/1
  egrmani/1 -> Gain2/1
  mVMANI1/1 -> MinMax/2
  Sum1/1 -> MinMax/1
  mVMANI2/1 -> Sum1/2
  vmani/1 -> Sum1/1
  airmani/1 -> Gain1/1
  MinMax/1 -> Product5/1
  Product5/1 -> MinMax3/2  "tmp_pmani"
  Product6/1 -> Product5/2
  constant1/1 -> Sum/2
  Sum/1 -> Product6/1
  tanmnp/1 -> Sum/1

== system AEMS_Standard_Library/SPECIFIC/AEMS_AS_PADE/A_pade_model ==
  Filter_param : Inport
  Vxx_in : Inport  Port=2
  Vxx_dly_t : Inport  Port=3
  Vbx_dly_init_ena : Inport  Port=4
  AEMS_FIRST_ORDER_FILTER_RST : AEMS_Standard_Library/FILTER/AEMS_FIRST_ORDER_FILTER_RST  Tag=[LIB]
      settings: AttributesFormatString=%<MaskType>
  A_filter_pade : Subsystem
  Vxx_in_dly : Outport
  Vxx_in_fil : Outport  Port=2
  wires:
  Vxx_dly_t/1 -> A_filter_pade/2(Vxx_dly_t)
  AEMS_FIRST_ORDER_FILTER_RST/1 -> Vxx_in_fil/1, A_filter_pade/1(Vxx_in_fil)
  Vxx_in/1 -> AEMS_FIRST_ORDER_FILTER_RST/3, AEMS_FIRST_ORDER_FILTER_RST/2
  A_filter_pade/1(Vxx_in_dly) -> Vxx_in_dly/1
  Vbx_dly_init_ena/1 -> AEMS_FIRST_ORDER_FILTER_RST/4, A_filter_pade/3(Vbx_dly_init_ena)
  Filter_param/1 -> AEMS_FIRST_ORDER_FILTER_RST/1
